simulink model "send_receive"  (Simulink 8.4)
settings: Solver=ode4  SolverMode=SingleTasking  StartTime=0.0  StopTime=inf  FixedStep=0.00005  MaxStep=0.01  RelTol=1e-3  AbsTol=1e-6
undefined symbols (not defined in the file): IP, UDP
libraries: rtlab x3, rtio_generic_ip x1
settings Model: Creator=jwu  LastModifiedBy=svo  ExtModeTrigMode=oneshot  ExtModeArmWhenConnect=off  BufferReuse=off
settings DataIOCC: ExternalInput=[]  InitialState=[]  LimitDataPoints=off  SaveOutput=off  SaveTime=off  SignalLoggingName=sigsOut
settings OptimizationCC: BooleanDataType=off  OptimizeBlockIOStorage=off  BufferReuse=off  GlobalBufferReuse=off  ExpressionFolding=off  FoldNonRolledExpr=off  LocalBlockOutputs=off  InitFltsAndDblsToZero=on
settings DebuggingCC: SaveWithParameterizedLinksMsg=none  SignalResolutionControl=TryResolveAllWithWarning  SolverPrmCheckMsg=none  InheritedTsInSrcMsg=none  MultiTaskDSMMsg=warning  MultiTaskCondExecSysMsg=none  StrictBusMsg=None
settings HardwareCC: TargetUnknown=on
settings RTWCC: IncludeERTFirstTime=on
settings CodeAppCC: IgnoreCustomStorageClasses=off
settings GRTTargetCC: TargetFcnLib=ansi_tfl_tmw.mat

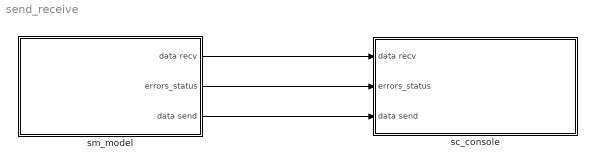
== system send_receive ==
  sc_console : Subsystem
  sm_model : Subsystem
  wires:
  sm_model/1(data recv) -> sc_console/1(data recv)
  sm_model/2(errors_status) -> sc_console/2(errors_status)
  sm_model/3(data send) -> sc_console/3(data send)

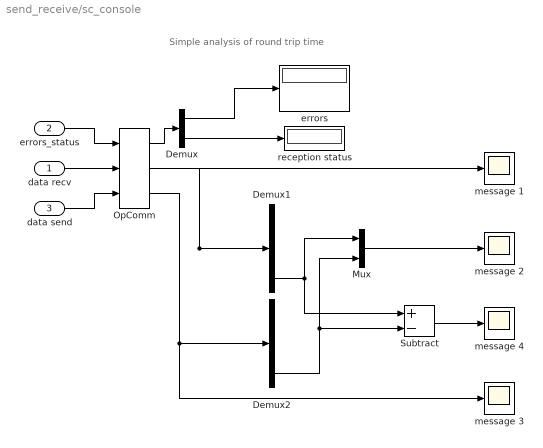
== system send_receive/sc_console ==
  note: Simple analysis of round trip time
  data recv : Inport
  errors_status : Inport  Port=2
  data send : Inport  Port=3
  Demux : Demux  Outputs=[2 1]
  Demux1 : Demux  Outputs=5
  Demux2 : Demux  Outputs=5
  Mux : Mux  Inputs=2
  OpComm : rtlab/OpComm  nbport=3  groupe_acq=1  subsys_rate=0  st=0  Synchronization=on  Interpolation=on  Threshold=1.0  Missed_Data=off  Sim_Time=off  Samples=off  dynSigOut=off  from_console=0  warning_done=off  writeOpCommFile=off  Offset=off
  Subtract : Sum  Inputs=+-
  errors : Display
  message {1..4} (4 alike) : Scope
      message 1 settings: YMin=-1.75  YMax=4
      message 2 settings: YMin=-1.75  YMax=4
      message 3 settings: YMin=-1.75  YMax=4  SaveName=ScopeData2
      message 4 settings: YMin=-1.75  YMax=4  SaveName=ScopeData3
  reception status : Display
  wires:
  errors_status/1 -> OpComm/1
  OpComm/2 -> Demux1/1, message 1/1
  data recv/1 -> OpComm/2
  OpComm/1 -> Demux/1
  Demux/1 -> errors/1
  Demux/2 -> reception status/1
  Mux/1 -> message 2/1
  data send/1 -> OpComm/3
  OpComm/3 -> Demux2/1, message 3/1
  Subtract/1 -> message 4/1
  Demux2/5 -> Mux/2, Subtract/2
  Demux1/5 -> Mux/1, Subtract/1

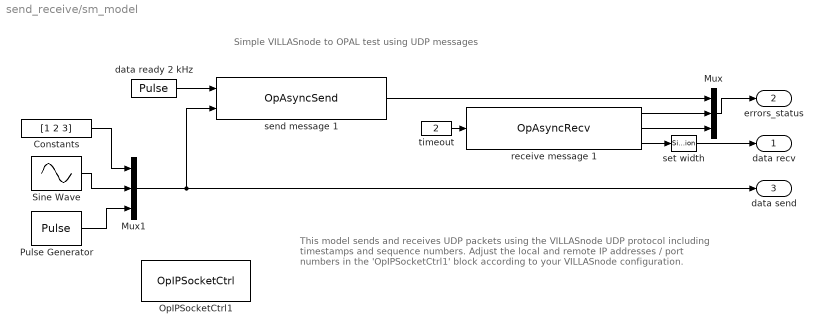
== system send_receive/sm_model ==
  note: This model sends and receives UDP packets using the VILLASnode UDP protocol
      | including timestamps and sequence numbers.
      |
      | Adjust the local and remote IP addresses / port numbers in the 'OpIPSocketCtrl1'
      | block according to your VILLASnode configuration.
  note: Simple VILLASnode to OPAL test using UDP messages
  Constants : Constant  Value=[1 2 3]
  Mux : Mux  Inputs=3
  Mux1 : Mux  Inputs=3
  OpIPSocketCtrl1 : rtio_generic_ip/OpIPSocketCtrl  ctl_id=1  proto=UDP/IP  ip_addr_remote=134.130.169.32  ip_port_remote=12008  ip_port_local=12008  ip_addr_mcast=0.0.0.0  exe_name=AsyncIP
  Pulse Generator : DiscretePulseGenerator  PulseType=Time based  Amplitude=5  Period=0.1  PulseWidth=30
  Sine Wave : Sin  Frequency=50*2*pi  SampleTime=0
  data ready 2 kHz : DiscretePulseGenerator  Period=10  SampleTime=0.00005
  receive message 1 : rtlab/Communication/Asynchronous/OpAsyncRecv  ctl_id=1  recv_id=1  enable_param=off  fp1=1  fp2=2  fp3=3  fp4=4  fp5=5  sp1=string1  sp2=string2  sp3=string3  sp4=string4  sp5=string5
  send message 1 : rtlab/Communication/Asynchronous/OpAsyncSend  ctl_id=1  send_id=1  mode=DONT_NEED_REPLY  enable_param=off  fp1=1  fp2=2  fp3=3  fp4=4  fp5=5  sp1=string1  sp2=string2  sp3=string3  sp4=string4  sp5=string5
  set width : SignalSpecification  Dimensions=5
  timeout : Constant  Value=2
  data recv : Outport
  errors_status : Outport  Port=2
  data send : Outport  Port=3
  wires:
  receive message 1/3 -> set width/1
  receive message 1/1 -> Mux/2
  receive message 1/2 -> Mux/3
  timeout/1 -> receive message 1/1
  send message 1/1 -> Mux/1
  Mux/1 -> errors_status/1
  set width/1 -> data recv/1
  Constants/1 -> Mux1/1
  Mux1/1 -> send message 1/2, data send/1
  data ready 2 kHz/1 -> send message 1/1
  Pulse Generator/1 -> Mux1/3
  Sine Wave/1 -> Mux1/2
